simulink model "problem3"  (R2024b)
settings: Solver=VariableStepAuto  StartTime=0.0  StopTime=100  RelTol=1e-3
model workspace (MAT data in the model file):
  P0 = [10000  0; 0  10000]
  alpha_1 = 0.0952
  beta_1 = -0.9048
  lambda = 0.9
  theta0 = [0; 0]
settings Model: Creator=djd14  LastModifiedBy=djd14

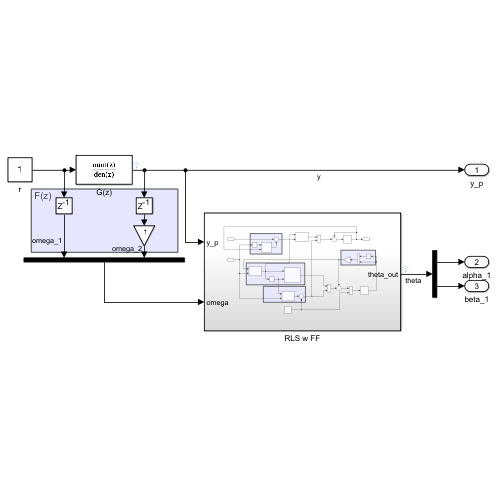
[thumbnail: Simulink's stored preview of the top-level diagram]
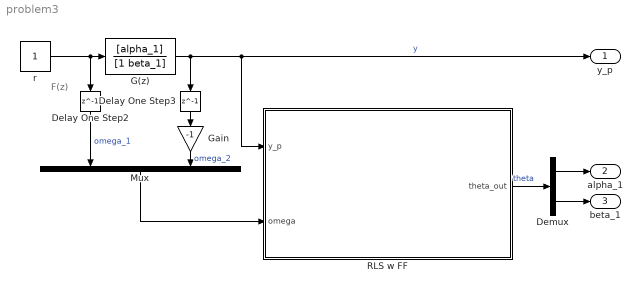
== system problem3 ==
  note: F(z)
  Delay One Step2 : Delay  DelayLength=1
  Delay One Step3 : Delay  DelayLength=1
  Demux : Demux  Outputs=2
  G(z) : DiscreteTransferFcn  Numerator=[alpha_1]  Denominator=[1 beta_1]
  Gain : Gain  Gain=-1
  Mux : Mux  Inputs=2
  RLS w FF : Subsystem
  r : Constant
  y_p : Outport  SampleTime=1
  alpha_1 : Outport  Port=2
  beta_1 : Outport  Port=3
  wires:
  r/1 -> G(z)/1, Delay One Step2/1
  Delay One Step2/1 -> Mux/1  "omega_1"
  Gain/1 -> Mux/2  "omega_2"
  Mux/1 -> RLS w FF/2(omega)
  G(z)/1 -> y_p/1, RLS w FF/1(y_p), Delay One Step3/1  "y"
  RLS w FF/1(theta_out) -> Demux/1  "theta"
  Demux/2 -> beta_1/1
  Demux/1 -> alpha_1/1
  Delay One Step3/1 -> Gain/1

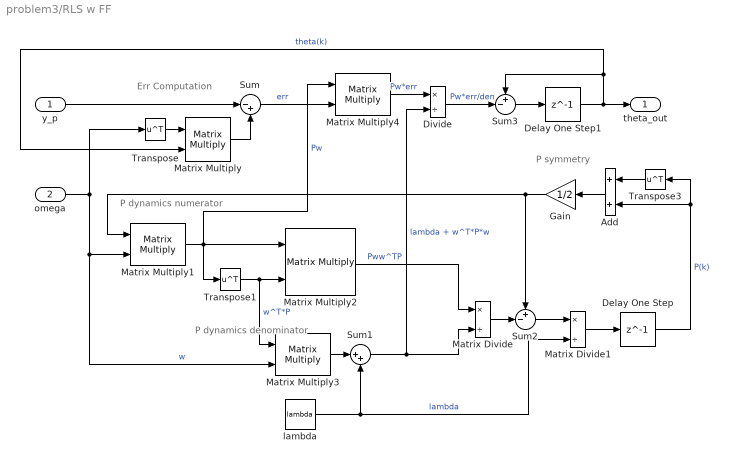
== system problem3/RLS w FF ==
  note: P symmetry
  note: P dynamics denominator
  note: P dynamics numerator
  note: Err Computation
  y_p : Inport
  omega : Inport  Port=2
  Add : Sum
  Delay One Step : Delay  DelayLength=1  InitialCondition=P0
  Delay One Step1 : Delay  DelayLength=1  InitialCondition=theta0
  Divide : Product  Inputs=*/
  Gain : Gain  Gain=1/2
  Matrix Divide : Product  Inputs=*/
  Matrix Divide1 : Product  Inputs=*/
  Matrix Multiply{,1..4} (5 alike) : Product  Multiplication=Matrix(*)
  Sum : Sum  Inputs=|-+
  Sum1 : Sum  Inputs=|++
  Sum2 : Sum  Inputs=+-|
  Sum3 : Sum  Inputs=+-|
  Transpose : Math  Operator=transpose
  Transpose1 : Math  Operator=transpose
  Transpose3 : Math  Operator=transpose
  lambda : Constant  Value=lambda
  theta_out : Outport
  wires:
  omega/1 -> Transpose/1, Matrix Multiply3/2, Matrix Multiply1/2  "w"
  Transpose/1 -> Matrix Multiply/1
  y_p/1 -> Sum/1
  Matrix Multiply/1 -> Sum/2
  Sum/1 -> Matrix Multiply4/2  "err"
  Matrix Multiply1/1 -> Matrix Multiply4/1, Matrix Multiply2/1, Transpose1/1  "Pw"
  Delay One Step/1 -> Transpose3/1, Add/2  "P(k)"
  Matrix Multiply2/1 -> Matrix Divide/1  "Pww^TP"
  Transpose1/1 -> Matrix Multiply3/1, Matrix Multiply2/2  "w^T*P"
  Matrix Multiply3/1 -> Sum1/1
  Sum1/1 -> Divide/2, Matrix Divide/2  "lambda + w^T*P*w"
  Matrix Divide/1 -> Sum2/2
  Sum2/1 -> Matrix Divide1/1
  Matrix Divide1/1 -> Delay One Step/1
  Transpose3/1 -> Add/1
  Add/1 -> Gain/1
  Gain/1 -> Matrix Multiply1/1, Sum2/1
  lambda/1 -> Matrix Divide1/2, Sum1/2  "lambda"
  Sum3/1 -> Delay One Step1/1
  Delay One Step1/1 -> theta_out/1, Matrix Multiply/2, Sum3/1  "theta(k)"
  Matrix Multiply4/1 -> Divide/1  "Pw*err"
  Divide/1 -> Sum3/2  "Pw*err/den"
